simulink model "Testing"  (R2024b)
settings: Solver=VariableStepAuto  StartTime=0.0  StopTime=75  RelTol=1e-3
libraries: SignalEditorBlockLib x1
settings Model: Creator=himma  LastModifiedBy=himma
settings DebuggingCC: AlgebraicLoopMsg=none

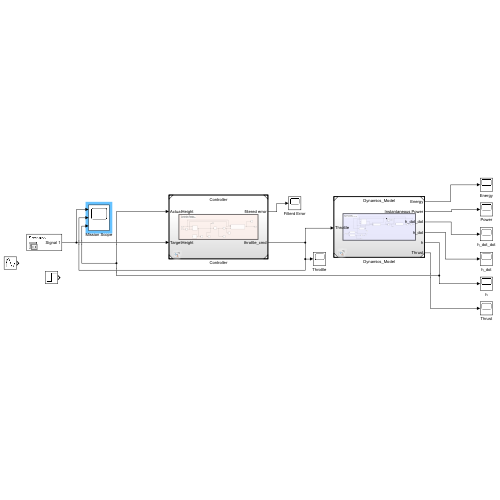
[thumbnail: Simulink's stored preview of the top-level diagram]
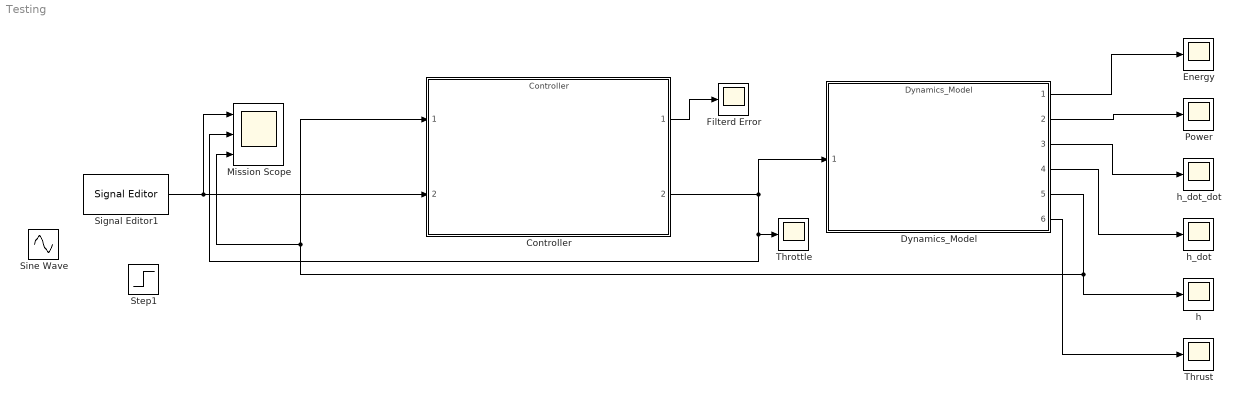
== system Testing ==
  Controller : ModelReference  ModelNameDialog=Controller.slx  SimulationMode=Normal  ModelReferenceVersion=1.15
  Dynamics_Model : ModelReference  ModelNameDialog=Dynamics_Model.slx  SimulationMode=Normal  ModelReferenceVersion=1.18
  Energy : Scope
  Filterd Error : Scope
  Mission Scope : Scope  NumInputPorts=3
  Power : Scope
  Signal Editor1 : SignalEditorBlockLib/Signal Editor  FileName=E:\EP2_Summer\Breif files\Simulink Testing (updated)\samplemission.mat  ActiveScenario=Scenario  ActiveSignal=Signal 1  IsBus=off  OutputBusObjectStr=Bus: BusObject  SampleTime=0.05  ZeroCross=off  OutputAfterFinalValue=Setting to zero  Unit=inherit  PreserveSignalName=on  ApplySigPropsToAllScenarios=on  ApplySigPropsToAllSignals=off
  Sine Wave : Sin  Amplitude=0.5  Bias=1  SampleTime=0
  Step1 : Step  Time=10  SampleTime=0.05
  Throttle : Scope
  Thrust : Scope
  h : Scope
  h_dot : Scope
  h_dot_dot : Scope
  wires:
  Signal Editor1/1 -> Controller/2, Mission Scope/1
  Dynamics_Model/5 -> Mission Scope/3, Controller/1, h/1
  Dynamics_Model/4 -> h_dot/1
  Dynamics_Model/3 -> h_dot_dot/1
  Dynamics_Model/2 -> Power/1
  Dynamics_Model/1 -> Energy/1
  Controller/1 -> Filterd Error/1
  Controller/2 -> Dynamics_Model/1, Mission Scope/2, Throttle/1
  Dynamics_Model/6 -> Thrust/1
